simulink model "Fourcarssimulink"  (R2022b)
settings: Solver=ode1  StartTime=0.0  StopTime=10.0  FixedStep=0.05  RelTol=1e-3
values from neighbouring files (symbols this model uses):
  Aol = sys_d.A    [fourcardynamics.m]
  Bol = sys_d.B    [fourcardynamics.m]
  Col = sys_d.C    [fourcardynamics.m]
  L_gain = (Aol*P*Col')/(Col*P*Col'+Rcov)    [fourcardynamics.m]
libraries: simulink x2
settings Model: Creator=Hp Business  LastModifiedBy=Hp Business

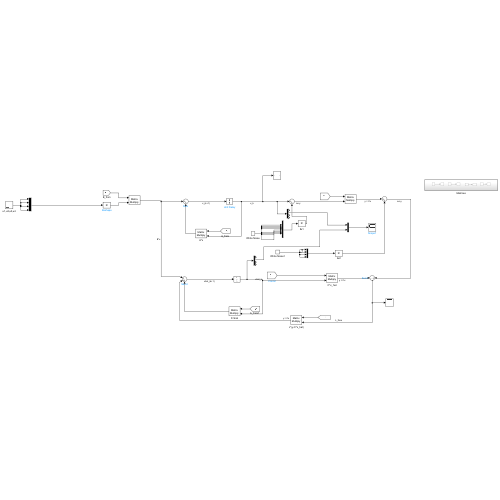
[thumbnail: Simulink's stored preview of the top-level diagram]
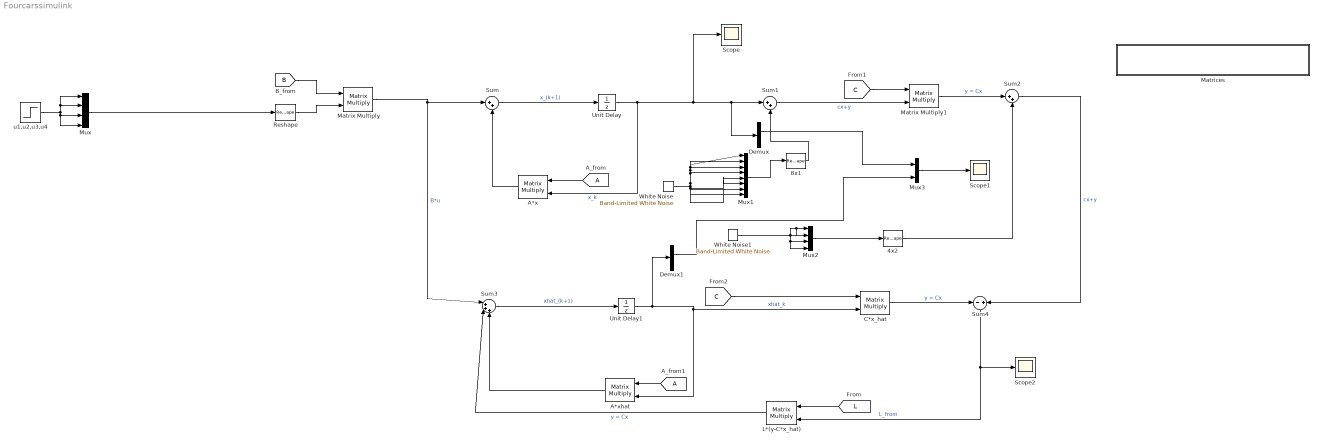
== system Fourcarssimulink ==
  4x2 : Reshape  OutputDimensionality=Customize  OutputDimensions=[4,1]
  8x1 : Reshape  OutputDimensionality=Customize  OutputDimensions=[8,1]
  A*x : Product  Multiplication=Matrix(*)
  A*xhat : Product  Multiplication=Matrix(*)
  A_from : From  TagVisibility=global
  A_from1 : From  TagVisibility=global
  C*x_hat : Product  Multiplication=Matrix(*)
  Demux : Demux
  Demux1 : Demux
  L*(y-C*x_hat) : Product  Multiplication=Matrix(*)
  Matrices : Subsystem
  Matrix Multiply : Product  Multiplication=Matrix(*)
  Matrix Multiply1 : Product  Multiplication=Matrix(*)
  Mux : Mux
  Mux1 : Mux  Inputs=8
  Mux2 : Mux
  Mux3 : Mux  Inputs=2
  Reshape : Reshape  OutputDimensionality=Customize  OutputDimensions=[4,1]
  Scope : Scope
  Scope1 : Scope
  Scope2 : Scope
  Sum : Sum  Inputs=|++
  Sum1 : Sum  Inputs=|++
  Sum2 : Sum  Inputs=|++
  Sum3 : Sum  Inputs=|+++
  Sum4 : Sum  Inputs=-+
  Unit Delay : UnitDelay  SampleTime=-1  HasFrameUpgradeWarning=on
  Unit Delay1 : UnitDelay  SampleTime=-1  HasFrameUpgradeWarning=on
  White Noise : simulink/Sources/Band-Limited White Noise  Cov=[0.1]  Ts=0.05  seed=[23341]
  White Noise1 : simulink/Sources/Band-Limited White Noise  Cov=[0.1]  Ts=0.05  seed=[23341]
  u1,u2,u3,u4 : Step  SampleTime=0
  wires:
  [B] -> Matrix Multiply/1
  Matrix Multiply/1 -> Sum/1, Sum3/1  "B*u"
  Sum/1 -> Unit Delay/1  "x_(k+1)"
  Unit Delay/1 -> Demux/1, Sum1/1, Scope/1, A*x/2  "x_k"
  A_from/1 -> A*x/1
  A*x/1 -> Sum/2
  Mux1/1 -> 8x1/1
  [C] -> Matrix Multiply1/1
  Mux2/1 -> 4x2/1
  White Noise1/1 -> Mux2/4, Mux2/3, Mux2/2, Mux2/1
  4x2/1 -> Sum2/2
  Matrix Multiply1/1 -> Sum2/1  "y = Cx"
  Sum2/1 -> Sum4/2  "cx+y"
  A_from1/1 -> A*xhat/1
  Unit Delay1/1 -> Demux1/1, C*x_hat/2, A*xhat/2  "xhat_k"
  Sum3/1 -> Unit Delay1/1  "xhat_(k+1)"
  A*xhat/1 -> Sum3/3
  [C] -> C*x_hat/1
  C*x_hat/1 -> Sum4/1  "y = Cx"
  Sum4/1 -> L*(y-C*x_hat)/2, Scope2/1  "L_from"
  [L] -> L*(y-C*x_hat)/1
  L*(y-C*x_hat)/1 -> Sum3/2  "y = Cx"
  Reshape/1 -> Matrix Multiply/2
  u1,u2,u3,u4/1 -> Mux/1, Mux/2, Mux/4, Mux/3
  Demux/2 -> Mux3/1
  Demux1/2 -> Mux3/2
  Mux3/1 -> Scope1/1
  8x1/1 -> Sum1/2
  White Noise/1 -> Mux1/5, Mux1/6, Mux1/8, Mux1/7, Mux1/1, Mux1/2, Mux1/3, Mux1/4
  Sum1/1 -> Matrix Multiply1/2  "cx+y"
  Mux/1 -> Reshape/1

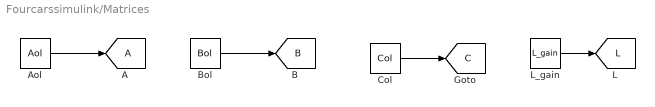
== system Fourcarssimulink/Matrices ==
  A : Goto  TagVisibility=global
  Aol : Constant  Value=Aol
  Bol : Constant  Value=Bol
  Col : Constant  Value=Col
  L_gain : Constant  Value=L_gain
  tag scope: B=global, C=global, L=global
  wires:
  Col/1 -> [C]
  L_gain/1 -> [L]
  Aol/1 -> A/1
  Bol/1 -> [B]
